simulink model "Prueba_ideal"  (R2020b)
settings: Solver=FixedStepAuto  StartTime=10  StopTime=25  FixedStep=0.001  RelTol=1e-3
settings Model: Creator=Tomas Tavella  LastModifiedBy=Tomas Tavella

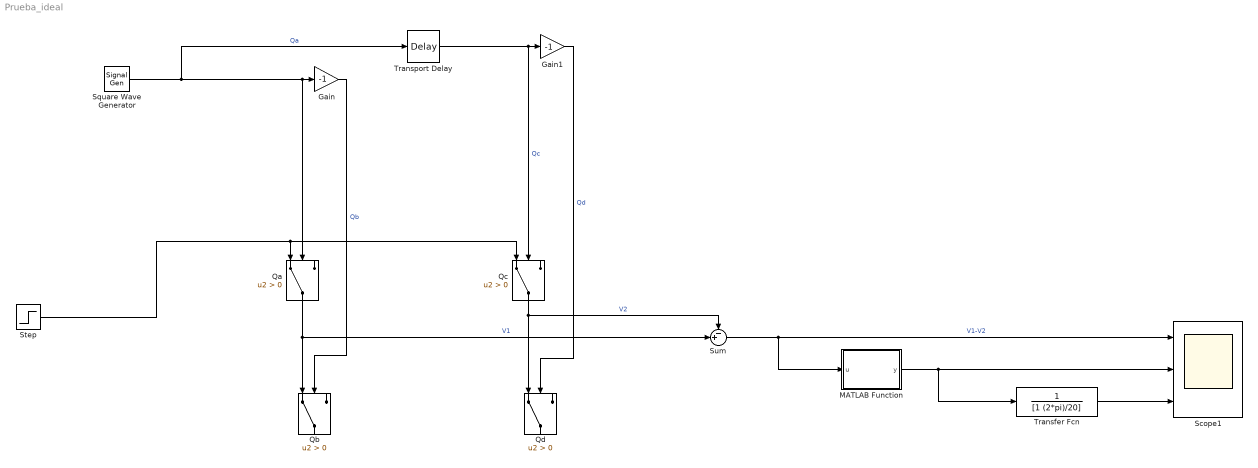
== system Prueba_ideal ==
  Gain : Gain  Gain=-1
  Gain1 : Gain  Gain=-1
  MATLAB Function : MATLAB Function  TreatAsAtomicUnit=on
  Qa : Switch  Criteria=u2 > Threshold
  Qb : Switch  Criteria=u2 > Threshold
  Qc : Switch  Criteria=u2 > Threshold
  Qd : Switch  Criteria=u2 > Threshold
  Scope1 : Scope  NumInputPorts=3
  Square Wave Generator : SignalGenerator  WaveForm=square
  Step : Step  Time=0.01  SampleTime=0
  Sum : Sum  Inputs=-+|
  Transfer Fcn : TransferFcn  Denominator=[1 (2*pi)/20]
  Transport Delay : TransportDelay  DelayTime=0.5
  wires:
  Square Wave Generator/1 -> Transport Delay/1, Qa/2, Gain/1  "Qa"
  Gain/1 -> Qb/2  "Qb"
  Transport Delay/1 -> Gain1/1, Qc/2  "Qc"
  Gain1/1 -> Qd/2  "Qd"
  Qa/1 -> Sum/2, Qb/1  "V1"
  Step/1 -> Qc/1, Qa/1
  Qc/1 -> Qd/1, Sum/1  "V2"
  Sum/1 -> MATLAB Function/1(u), Scope1/1  "V1-V2"
  MATLAB Function/1(y) -> Transfer Fcn/1, Scope1/2
  Transfer Fcn/1 -> Scope1/3

== matlab function Prueba_ideal/MATLAB Function ==
  data: u input; y output
function y = rect(u)
    
    if u>=0
        y = u;
    else
        y = -u;
    end
    
end
